simulink model "getEncoders"  (Simulink 7.9)
settings: Solver=ode45  StartTime=0.0  StopTime=inf  RelTol=1e-3
libraries: utility x1
settings Model: Creator=jorhabib  LastModifiedBy=jorhabib

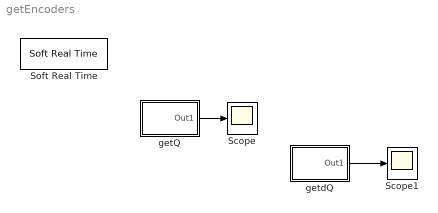
== system getEncoders ==
  Scope : Scope
      settings: YMin=-0.6  YMax=0.8  SampleTime=0.1
  Scope1 : Scope
      settings: YMin=-0.6  YMax=0.8  SampleTime=0.1
  Soft Real Time : utility/Soft Real Time  x=0.1
  getQ : Subsystem
  getdQ : Subsystem
  wires:
  getQ/1(Out1) -> Scope/1
  getdQ/1(Out1) -> Scope1/1

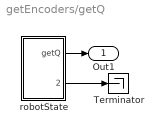
== system getEncoders/getQ ==
  Terminator : Terminator
  robotState : Subsystem
  Out1 : Outport
  wires:
  robotState/2(getDq) -> Terminator/1
  robotState/1(getQ) -> Out1/1

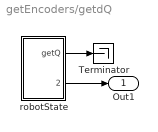
== system getEncoders/getdQ ==
  Terminator : Terminator
  robotState : Subsystem
  Out1 : Outport
  wires:
  robotState/1(getQ) -> Terminator/1
  robotState/2(getDq) -> Out1/1

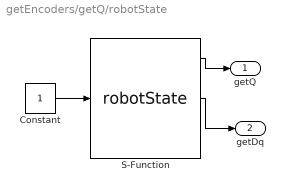
== system getEncoders/getQ/robotState ==
  Constant : Constant
  S-Function : S-Function  FunctionName=robotState  EnableBusSupport=off
  getQ : Outport
  getDq : Outport  Port=2
  wires:
  S-Function/1 -> getQ/1
  S-Function/2 -> getDq/1
  Constant/1 -> S-Function/1

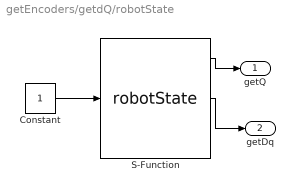
== system getEncoders/getdQ/robotState ==
  Constant : Constant
  S-Function : S-Function  FunctionName=robotState  EnableBusSupport=off
  getQ : Outport
  getDq : Outport  Port=2
  wires:
  S-Function/2 -> getDq/1
  S-Function/1 -> getQ/1
  Constant/1 -> S-Function/1
